simulink model "sesAgent"  (Simulink 6.2)
settings: Solver=ode45  StartTime=0.0  StopTime=10.0  RelTol=1e-3
settings Model: LastModifiedBy=achimk
settings DebuggingCC: SolverPrmCheckMsg=warning

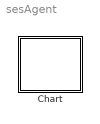
== system sesAgent ==
  Chart : Stateflow chart

== stateflow chart Chart ==
  state ProcessImgCalculateSESSalienceAndFindFOA
    \\Sally\LeftCameraAgent\FrameGrabber.ObtainImage()
    \\Sally\SESAGENT\SES.ProcessImage()
    \\Sally\SESAGENT\SES.CalculateSalience()
    \\Sally\SESAGENT\CopyVS.CopyCurrentVector()
    \\Sally\HeadAgent\PTControl.aaHeadCommand()
  state Initial
    \\Sally\LeftCameraAgent\FrameGrabber.Initialize()
    \\Sally\LeftCameraAgent\FrameGrabber.ObtainImage()
    \\Sally\LeftCameraAgent\FrameGrabber.ObtainImage()
    \\Sally\SESAGENT\SES.ResetSES()
  (default) -> Initial : Start
  Initial -> ProcessImgCalculateSESSalienceAndFindFOA : Always
  ProcessImgCalculateSESSalienceAndFindFOA -> ProcessImgCalculateSESSalienceAndFindFOA : Always
  data: headangles local double size=4
